simulink model "s_maglev_pi"  (Simulink 7.7)
settings: Solver=ode4  StartTime=0.0  StopTime=10  FixedStep=0.002  RelTol=1e-3
values from neighbouring files (symbols this model uses):
  IC_MAX = 3    [config_maglev.m]
  Ki_c = wn_c^2 * tau_c / Kc_dc    [d_maglev_pi_piv.m]    (also in setup_maglev.m = 0)
  Kp_c = (2*zeta_c*wn_c*tau_c - 1) / Kc_dc    [d_maglev_pi_piv.m]    (also in setup_maglev.m = 0)
  Lc = 0.4125    [config_maglev.m]
  Rc = 10    [config_maglev.m]
  Rs = 1    [config_maglev.m]
  VMAX_AMP = 24    [config_maglev.m]
settings Model: Creator=MLevis  LastModifiedBy=MLevis  ExtModeTrigDuration=5000
settings SolverCC: PositivePriorityOrder=on
settings RTWCC: SystemTargetFile=quarc_win64.tlc  TemplateMakefile=quarc_default_tmf  Description=QUARC Win64 Target  ProcessScript=quarc_win64_make_rtw_hook
settings STFCustomTargetCC: TargetPreCompLibLocation=C:\PROGRA~3\QUARC\lib\2011a\win64\release  FunctionExecutionProfile=off  GeneratePreprocessorConditionals=Disable all  SystemTargetFile=quarc_win64.tlc
settings GRTTargetCC: TargetPreCompLibLocation=C:\PROGRA~3\QUARC\lib\2011a\win64\release  ParMdlRefBuildCompliant=off  CompOptLevelCompliant=off  MatFileLogging=off  ExtMode=on  ExtModeMexFile=quarc_comm

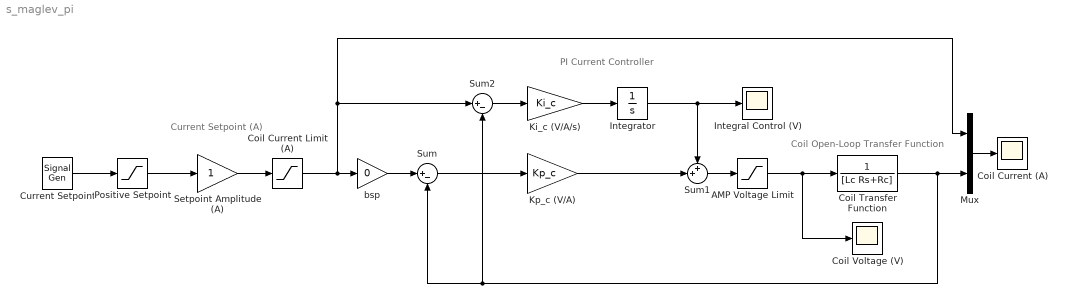
== system s_maglev_pi ==
  note: Current Setpoint (A)
  note: PI Current Controller
  note: Coil Open-Loop
      | Transfer Function
  AMP Voltage Limit : Saturate  UpperLimit=VMAX_AMP  LowerLimit=-VMAX_AMP
  Coil Current Limit (A) : Saturate  UpperLimit=IC_MAX  LowerLimit=0
  Coil Current (A) : Scope
      settings: TimeRange=10  YMin=-0.5  YMax=2.5  SaveName=data_Ic  DataFormat=Array
  Coil Transfer Function : TransferFcn  Denominator=[Lc Rs+Rc]
  Coil Voltage (V) : Scope
      settings: TimeRange=10  YMax=25  SaveName=data_Vc  DataFormat=Array
  Current Setpoint : SignalGenerator  WaveForm=square  Frequency=.2
  Integral Control (V) : Scope
      settings: TimeRange=10  YMin=-50  YMax=300  SaveName=data_Vc1  DataFormat=Array
  Integrator : Integrator  UpperSaturationLimit=VMAX_AMP  LowerSaturationLimit=-VMAX_AMP
  Ki_c (V/A/s) : Gain  Gain=Ki_c  SaturateOnIntegerOverflow=on  OutDataTypeStr=Inherit: Same as input  ParamDataTypeStr=Inherit: Same as input
  Kp_c (V/A) : Gain  Gain=Kp_c  SaturateOnIntegerOverflow=on  OutDataTypeStr=Inherit: Same as input  ParamDataTypeStr=Inherit: Same as input
  Mux : Mux  Inputs=2
  Positive Setpoint : Saturate  UpperLimit=1  LowerLimit=0
  Setpoint Amplitude (A) : Gain  SaturateOnIntegerOverflow=on  OutDataTypeStr=Inherit: Same as input  ParamDataTypeStr=Inherit: Same as input
  Sum : Sum  Inputs=|+-
  Sum1 : Sum  Inputs=++|
  Sum2 : Sum  Inputs=|+-
  bsp : Gain  Gain=0
  wires:
  Current Setpoint/1 -> Positive Setpoint/1
  Setpoint Amplitude (A)/1 -> Coil Current Limit (A)/1
  Coil Current Limit (A)/1 -> Mux/1, Sum2/1, bsp/1
  Kp_c (V/A)/1 -> Sum1/2
  Coil Transfer Function/1 -> Mux/2, Sum/2, Sum2/2
  Mux/1 -> Coil Current (A)/1
  Positive Setpoint/1 -> Setpoint Amplitude (A)/1
  Sum1/1 -> AMP Voltage Limit/1
  Sum2/1 -> Ki_c (V/A/s)/1
  bsp/1 -> Sum/1
  Sum/1 -> Kp_c (V/A)/1
  Ki_c (V/A/s)/1 -> Integrator/1
  Integrator/1 -> Sum1/1, Integral Control (V)/1
  AMP Voltage Limit/1 -> Coil Transfer Function/1, Coil Voltage (V)/1
